simulink model "Prescan_Carsim_0118_cs_old"  (R2019b)
settings: Solver=ode5  StartTime=0.0  StopTime=inf  FixedStep=1/1000  RelTol=1e-3
PreLoadFcn:
  | mbxruntime.callbacks.PreLoadFcn(bdroot);
PostLoadFcn:
  | mbxruntime.callbacks.PostLoadFcn(bdroot);
InitFcn:
  | mbxruntime.callbacks.InitFcn(bdroot);
  | Initialization_Func;
  | %T01_Init_2106;
StartFcn:
  | mbxruntime.callbacks.StartFcn(bdroot);
  | current_sys=gcs;
  | speedblock=Simulink.findBlocks(current_sys,'Name','speed_kmh_Gain');
  | h1=add_exec_event_listener(speedblock,'PostOutputs',@SpeedVisulization);
  | outblock=Simulink.findBlocks(current_sys,'Name','trajectorycurveoutput_Gain');
  | CurveTrajectoryListenerHandle=add_exec_event_listener(outblock,'PostOutputs',@TrajectoryCurve_CallBack);
  | lanedatablock=Simulink.findBlocks(current_sys,'Name','LaneData_Gain');
  | CurveLaneListenerHandle=add_exec_event_listener(lanedatablock,'PostOutputs',@CurveLane_CallBack);
StopFcn:
  | mbxruntime.callbacks.StopFcn(bdroot);
model workspace: external: MAT-File .\Prescan_Carsim_0118_cs_hws.mat (data not in the file)
values from neighbouring files (symbols this model uses):
  g = 9.8    [Initialization_Func.m]
  InitialPlanningParameter = [0,0,1,0,2,2,2,40,60]'    [Initialization_Func.m]
  Kf = 20000    [Initialization_Func.m]
  Kr = 20000    [Initialization_Func.m]
  Lr = 1.644    [Initialization_Func.m]
  M = 1275    [Initialization_Func.m]
  nG = 24    [Initialization_Func.m]
  V = 60/3.6    (= 16.6666666667)    [Initialization_Func.m]
  VehicleBaseLength = Lf+Lr    (= 2.66)    [Initialization_Func.m]
undefined symbols (not defined in the file or in its folder): AAx, AAy, AAz, AVx, AVy, AVz, Ax, Ay, Az, canChannel, DiscIntNeverNeededParam, InitialDPMPDF_Comfort, InitialDPMPDF_Efficiency, InitialDPMPDF_Safety, InitialPDF_DEM, mbxruntime, NormalisedTrajectoryIndicator_Pool, Parameter_Indicator_LookUpTable, Prescan_Carsim_1230_cs_0658e9ca1334a8be, Prescan_Carsim_1230_cs_08c5eb9a1bd7376a, Prescan_Carsim_1230_cs_6cfd759b89b9fc85, Prescan_Carsim_1230_cs_9435cc1cceb5050d, Prescan_Carsim_1230_cs_ac716d34d49f74ab, Prescan_Carsim_1230_cs_be02757d7f212dd5, Rational_Coefficient_Learning, SteeringWheel, TrajectoryIndicatorRange, Vx, Vy, Vz, WheelL0, WheelL1, WheelR0, WheelR1
libraries: canmsglib x11, dsparch4 x6, canlib x3, PreScanSimulinkLibrary x3, Solver_SF x1, autolibshared x1
(part 3 of 8)

== system Prescan_Carsim_0118_cs_old/BMW_X5_SUV_1/Connect The Target /simplefilter ==
  In1 : Inport
  Add : Sum
  Gain : Gain  Gain=0.5
  Memory : Memory
  Out1 : Outport  VectorParamsAs1DForOutWhenUnconnected=off
  wires:
  Gain/1 -> Out1/1
  Memory/1 -> Add/2
  Add/1 -> Gain/1
  In1/1 -> Memory/1, Add/1

== system Prescan_Carsim_0118_cs_old/BMW_X5_SUV_1/DEM updating and Preference Estimation/UpdateDEM ==
  FeedBack_FromDriver : Inport
  TrajectoryIndicator : Inport  Port=2
  Trigger : TriggerPort  TriggerType=either  VariantControl=Variant  PortDimensions=1
  Constant1 : Constant  Value=InitialPDF_DEM
      settings: AttributesFormatString=|
      | The Initial probability density Distribution
      | of the S-C-E weight of the DEM
  Constant2 : Constant  Value=InitialDPMPDF_Safety
      settings: AttributesFormatString=|
      | The Initial probability density Distribution
      | of the DPM for S-C-E
  Constant5 : Constant  Value=InitialDPMPDF_Comfort
      settings: AttributesFormatString=|
      | The Initial probability density Distribution
      | of the DPM for S-C-E
  Constant6 : Constant  Value=InitialDPMPDF_Efficiency
      settings: AttributesFormatString=|
      | The Initial probability density Distribution
      | of the DPM for S-C-E
  Construct Comparison Group : Subsystem
  Online DEM updating : Subsystem
  Trajectory Planning Parameter Management1 : Subsystem  Commented=on
  Trajectory Planning Parameter Management2 : Subsystem
  online DPM building preference estimation accordign to feedback : Subsystem  Commented=on
  PlanningParameter : Outport  InitialOutput=InitialPlanningParameter
  Expected_QueryID : Outport  Port=2
  wires:
  Construct Comparison Group/1(FeedBack) -> Online DEM updating/1(FeedBack)
  online DPM building preference estimation accordign to feedback/1(Expected_TrajectoryIndicators) -> Trajectory Planning Parameter Management1/1(Expected_TrajectoryIndicators)
  online DPM building preference estimation accordign to feedback/2(ExpectedNext_QueryID) -> Trajectory Planning Parameter Management1/2(ExpectedNext_QueryID)
  Trajectory Planning Parameter Management2/1(Trajectory parameter) -> PlanningParameter/1
  Online DEM updating/1(Next_ExpectedTrajectoryIndicator) -> Trajectory Planning Parameter Management2/1(Expected_TrajectoryIndicators)
  Construct Comparison Group/2(Query_Normalized) -> Online DEM updating/2(Query_Compare)
  Constant2/1 -> Online DEM updating/4(PriorDPMPDF_Safety)
  Constant1/1 -> Online DEM updating/3(PriorPDF_DEM)
  Constant6/1 -> Online DEM updating/6(PriorDPMPDF_Efficiency)
  Online DEM updating/2(Next_ExpectedTrajectoryID) -> Trajectory Planning Parameter Management2/2(Next_ExpectedTrajectoryIndicatorID), Expected_QueryID/1
  Constant5/1 -> Online DEM updating/5(PriorDPMPDF_Comfort)
  Construct Comparison Group/3(Evaluated_NormlisedTrajectoryIndicator) -> Online DEM updating/7(Evaluated_Normalised)
  Construct Comparison Group/4(LastPreference_Normalised) -> Online DEM updating/8(LastPreference_NormalisedTrajectoryIndicator)
  FeedBack_FromDriver/1 -> Construct Comparison Group/1(FeedBack_FromDriver)
  TrajectoryIndicator/1 -> Construct Comparison Group/2(TrajectoryIndicator)

== system Prescan_Carsim_0118_cs_old/BMW_X5_SUV_1/DriverFeedBack/Generate the FeedBack Obtainment Trigger Signal ==
  CurveFlag : Inport
  Add : Sum  Inputs=-+
  Clock : Clock
  ConsideringTime (s) : Constant  Value=2
  Relational Operator : RelationalOperator  Operator=>  OutDataTypeStr=boolean  RndMeth=Simplest
  Subsystem : Subsystem
  Trigger Signal of Feedback obtainement : Outport
  wires:
  ConsideringTime (s)/1 -> Relational Operator/2
  Add/1 -> Relational Operator/1  "CurveTime"
  Clock/1 -> Add/2, Subsystem/1(In1)
  Subsystem/1(Beginning Time) -> Add/1
  CurveFlag/1 -> Subsystem/Trigger
  Relational Operator/1 -> Trigger Signal of Feedback obtainement/1

== system Prescan_Carsim_0118_cs_old/BMW_X5_SUV_1/DriverFeedBack/driver evaluation model ==
  TrajectoryIndicators : Inport
  Trigger : TriggerPort  VariantControl=Variant  PortDimensions=1
  Constant : Constant
      settings: AttributesFormatString=|
      | 1: "complete_rational"
      | 2: "probability_rational"
      | 3: "bound_rational"
  RationalCoefficient_Sim : Constant  Value=5
  Scope : Scope
  SimPreferenceDPM_Comfort : Constant  Value=[1,1]
  SimPreferenceDPM_Efficiency : Constant  Value=[1,1]
  SimPreferenceDPM_Safety : Constant  Value=[1,1]
  SimPreference_DEM : Constant  Value=[0.3,0.4,0.3]
  Simulated Driver : MATLAB Function  TreatAsAtomicUnit=on
  feedback : Outport
      settings: AttributesFormatString=|
      | 0: There is no comparison
      | 1: Prefer the former one
      | 2：Prefer the latter one
      | 3: No obvious preference
  FeedBack_Trigger : Outport  Port=2
  wires:
  Simulated Driver/1(Compare_Result) -> feedback/1
  Simulated Driver/3(mis_answered_ind) -> Scope/1
  SimPreference_DEM/1 -> Simulated Driver/2(Preference_DEM)
  SimPreferenceDPM_Safety/1 -> Simulated Driver/3(PreferenceDPM_Safety)
  SimPreferenceDPM_Comfort/1 -> Simulated Driver/4(PreferenceDPM_Comfort)
  SimPreferenceDPM_Efficiency/1 -> Simulated Driver/5(PreferenceDPM_Efficiency)
  RationalCoefficient_Sim/1 -> Simulated Driver/6(Rational_coefficient)
  Constant/1 -> Simulated Driver/7(Driver_Type)
  TrajectoryIndicators/1 -> Simulated Driver/1(TrajectoryIndicator)
  Simulated Driver/2(FeedBack_Count) -> FeedBack_Trigger/1

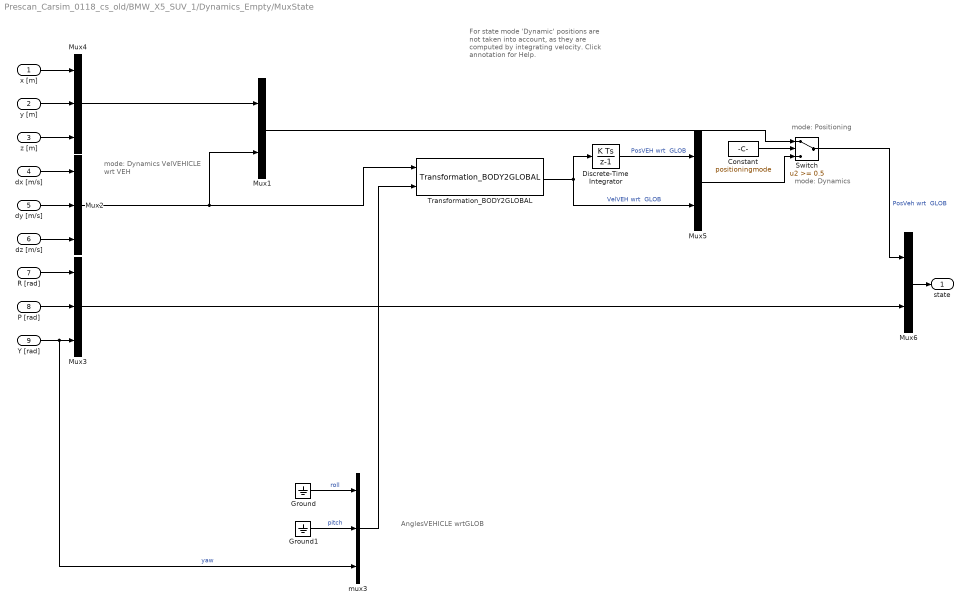
== system Prescan_Carsim_0118_cs_old/BMW_X5_SUV_1/Dynamics_Empty/MuxState ==
  note: mode: Dynamics
  note: mode: Positioning
  note: mode: Dynamics
      | VelVEHICLE
      | wrt VEH
  note: AnglesVEHICLE
      | wrtGLOB
  note: For state mode 'Dynamic' positions
      | are not taken into account, as they
      | are computed by integrating velocity.
      | Click annotation for Help.
  x [m] : Inport  SampleTime=TimeStep
  y [m] : Inport  Port=2  SampleTime=TimeStep
  z [m] : Inport  Port=3  SampleTime=TimeStep
  dx [m/s] : Inport  Port=4  SampleTime=TimeStep
  dy [m/s] : Inport  Port=5  SampleTime=TimeStep
  dz [m/s] : Inport  Port=6  SampleTime=TimeStep
  R [rad] : Inport  Port=7  SampleTime=TimeStep
  P [rad] : Inport  Port=8  SampleTime=TimeStep
  Y [rad] : Inport  Port=9  SampleTime=TimeStep
  Constant : Constant  DisableCoverage=on  Value=positioningmode
  Discrete-Time Integrator : DiscreteIntegrator  SampleTime=TimeStep  ICPrevOutput=DiscIntNeverNeededParam  ICPrevScaledInput=DiscIntNeverNeededParam
  Ground : Ground
  Ground1 : Ground
  Mux1 : Mux  Inputs=[3 3]
  Mux2 : Mux  Inputs=3
  Mux3 : Mux  Inputs=3
  Mux4 : Mux  Inputs=3
  Mux5 : Mux  Inputs=[3 3]
  Mux6 : Mux  Inputs=[6 3]
  Switch : Switch  Threshold=0.5
  Transformation_BODY2GLOBAL : PreScanSimulinkLibrary/Simple_Vehicle_Dynamics/Chassis/MuxDynState/Transformation_BODY2GLOBAL  SystemSampleTime=-1  Latency=0  AutoFrameSizeCalculation=off
  mux3 : Mux  Inputs=3
  state : Outport
  wires:
  Constant/1 -> Switch/2
  Mux6/1 -> state/1
  Mux4/1 -> Mux1/1
  Mux5/1 -> Switch/3
  Mux1/1 -> Switch/1
  Switch/1 -> Mux6/1  "PosVeh wrt  GLOB"
  P [rad]/1 -> Mux3/2
  R [rad]/1 -> Mux3/1
  dz [m/s]/1 -> Mux2/3
  dy [m/s]/1 -> Mux2/2
  dx [m/s]/1 -> Mux2/1
  z [m]/1 -> Mux4/3
  y [m]/1 -> Mux4/2
  x [m]/1 -> Mux4/1
  Ground1/1 -> mux3/2  "pitch"
  Y [rad]/1 -> mux3/3, Mux3/3  "yaw"
  Mux3/1 -> Mux6/2
  Transformation_BODY2GLOBAL/1 -> Discrete-Time Integrator/1, Mux5/2  "VelVEH wrt  GLOB"
  mux3/1 -> Transformation_BODY2GLOBAL/2
  Ground/1 -> mux3/1  "roll"
  Mux2/1 -> Mux1/2, Transformation_BODY2GLOBAL/1
  Discrete-Time Integrator/1 -> Mux5/1  "PosVEH wrt  GLOB"

== system Prescan_Carsim_0118_cs_old/BMW_X5_SUV_1/Dynamics_Empty/STATE_BMW_X5_SUV_1 ==
  State : Inport  SampleTime=TimeStep
  Bus Creator : BusCreator  Inputs=15  OutDataTypeStr=Bus: PRESCAN_STATEACTUATORDATA  NonVirtualBus=on
  Constant : Constant  Value=0
  Demux : Demux  Outputs=15
  Mux : Mux  Inputs=3
  Mux1 : Mux  Inputs=3
  Mux2 : Mux  Inputs=3
  iniBODYAngles wrtVEH [rad] : Constant  Value=Roll0  SampleTime=TimeStep
  iniBODYAngles wrtVEH [rad]1 : Constant  Value=Pitch0  SampleTime=TimeStep
  iniVEHAngles wrtGLOB [rad] : Constant  Value=Yaw0  SampleTime=TimeStep
  iniVEHposition wrtGLOB [m] : Constant  Value=x0  SampleTime=TimeStep
  iniVEHposition wrtGLOB [m]1 : Constant  Value=y0  SampleTime=TimeStep
  iniVEHposition wrtGLOB [m]2 : Constant  Value=z0  SampleTime=TimeStep
  state2FullState : PreScanSimulinkLibrary/state2FullState  SystemSampleTime=-1  Latency=0  AutoFrameSizeCalculation=off
  StateBus : Outport  OutDataTypeStr=Bus: PRESCAN_STATEACTUATORDATA
  wires:
  Mux2/1 -> state2FullState/4
  iniVEHAngles wrtGLOB [rad]/1 -> Mux2/3
  Mux1/1 -> state2FullState/3
  Constant/1 -> Mux2/1, Mux2/2, Mux1/3
  iniBODYAngles wrtVEH [rad]1/1 -> Mux1/2
  iniBODYAngles wrtVEH [rad]/1 -> Mux1/1
  Mux/1 -> state2FullState/2
  iniVEHposition wrtGLOB [m]2/1 -> Mux/3
  iniVEHposition wrtGLOB [m]/1 -> Mux/1
  iniVEHposition wrtGLOB [m]1/1 -> Mux/2
  Demux/15 -> Bus Creator/15  "AngularVelocityYaw"
  Demux/14 -> Bus Creator/14  "AngularVelocityPitch"
  Demux/13 -> Bus Creator/13  "AngularVelocityRoll"
  Demux/12 -> Bus Creator/12  "OrientationYaw"
  Demux/11 -> Bus Creator/11  "OrientationPitch"
  Demux/10 -> Bus Creator/10  "OrientationRoll"
  Demux/9 -> Bus Creator/9  "AccelerationZ"
  Demux/8 -> Bus Creator/8  "AccelerationY"
  Demux/7 -> Bus Creator/7  "AccelerationX"
  Demux/6 -> Bus Creator/6  "VelocityZ"
  Demux/5 -> Bus Creator/5  "VelocityY"
  Demux/4 -> Bus Creator/4  "VelocityX"
  Demux/3 -> Bus Creator/3  "PositionZ"
  Demux/2 -> Bus Creator/2  "PositionY"
  Demux/1 -> Bus Creator/1  "PositionX"
  state2FullState/1 -> Demux/1
  State/1 -> state2FullState/1
  Bus Creator/1 -> StateBus/1

== system Prescan_Carsim_0118_cs_old/BMW_X5_SUV_1/SELF_Demux/compas converter ==
  rotz [rad] : Inport
  cart2compas : Subsystem
  rad2deg : Gain  Gain=180/pi
  heading [deg] : Outport
  wires:
  rad2deg/1 -> cart2compas/1(Angle [deg])
  rotz [rad]/1 -> rad2deg/1
  cart2compas/1(heading [deg]) -> heading [deg]/1

== system Prescan_Carsim_0118_cs_old/BMW_X5_SUV_1/Tracking Control & vehicle dynamics/Lane Keeping Assistance ==
  note: Trajectory Trackin-LQR controller, Carsim Model
  note: Trajectory Trackin-LQR controller, Simulink VDM
  note: Trajectory Tracking Controller-SMC controller
  DataUsedForTracking (PrescanToTarget)t : Inport
  Bus Selector : BusSelector  OutputSignals=Preview Error,HeadError_rad,Curvature,PreviewDistance,Speed_Kmh
  Digital Filter Design6 : dsparch4/Digital Filter Design  Commented=on  mwdsp_browser_bugfix_var=off
  From : From  Commented=on  GotoTag=SMC_c1  TagVisibility=global
  From1 : From  Commented=on  GotoTag=SMC_c2  TagVisibility=global
  From3 : From  Commented=on  GotoTag=delta  TagVisibility=global
  From4 : From  Commented=on  GotoTag=kapa  TagVisibility=global
  Gain : Gain  Gain=180/pi
  Gain1 : Gain  Gain=1/3.6
  Manual Switch : ManualSwitch  CurrentSetting=0
  Manual Switch1 : ManualSwitch  CurrentSetting=0
  Path Tracking - LQR controller : Subsystem  Commented=on
  Path Tracking - LQR controller1 : Subsystem
  Path Tracking - SMC controller : MATLAB Function  Commented=on  TreatAsAtomicUnit=on
  SMC characters : Subsystem  Commented=on
  derivative_filter : Subsystem
  "derivative_filter " : Subsystem
  steering angle_Front(deg) : Outport
  wires:
  Path Tracking - LQR controller/1(SteeringAngle_Front(rad)) -> Manual Switch1/1
  Gain1/1 -> Path Tracking - LQR controller1/7(Speed_m/s), Path Tracking - LQR controller/7(Speed_m/s), Path Tracking - SMC controller/11(v)
  Gain/1 -> steering angle_Front(deg)/1
  "derivative_filter "/1(Out1) -> Path Tracking - LQR controller1/2(PreviewError_dot), Path Tracking - LQR controller/2(PreviewError_dot), Path Tracking - SMC controller/6(PreviewError_dot)
  Digital Filter Design6/1 -> Manual Switch/1  "steering angle"
  From/1 -> Path Tracking - SMC controller/1(c1)
  derivative_filter/1(Out1) -> Path Tracking - LQR controller1/4(HeadingError_dot), Path Tracking - LQR controller/4(HeadingError_dot), Path Tracking - SMC controller/8(HeadingError_dot)
  Path Tracking - SMC controller/1(SteerAngle) -> Digital Filter Design6/1
  From3/1 -> Path Tracking - SMC controller/3(delta)
  From1/1 -> Path Tracking - SMC controller/2(c2)
  From4/1 -> Path Tracking - SMC controller/4(kapa)
  Bus Selector/5 -> Gain1/1  "<Speed_Kmh>"
  Bus Selector/1 -> Path Tracking - SMC controller/5(PreviewError), Path Tracking - LQR controller1/1(PreviewError), Path Tracking - LQR controller/1(PreviewError), "derivative_filter "/1(In1)  "<Preview Error>"
  Bus Selector/4 -> Path Tracking - SMC controller/10(PreviewDistance), Path Tracking - LQR controller1/6(Preview_Distance), Path Tracking - LQR controller/6(Preview_Distance)  "<PreviewDistance>"
  Bus Selector/2 -> Path Tracking - LQR controller1/3(HeadingError), Path Tracking - LQR controller/3(HeadingError), Path Tracking - SMC controller/7(HeadingError), derivative_filter/1(In1)  "<HeadError_rad>"
  Manual Switch/1 -> Gain/1
  Bus Selector/3 -> Path Tracking - LQR controller1/5(Curvature), Path Tracking - LQR controller/5(Curvature), Path Tracking - SMC controller/9(Curvature)  "<Curvature>"
  DataUsedForTracking (PrescanToTarget)t/1 -> Bus Selector/1
  Path Tracking - LQR controller1/1(SteeringAngle_Front(rad)) -> Manual Switch1/2
  Manual Switch1/1 -> Manual Switch/2

== system Prescan_Carsim_0118_cs_old/BMW_X5_SUV_1/Tracking Control & vehicle dynamics/simple_filter10 ==
  In1 : Inport
  Add : Sum
  Gain10 : Gain  Gain=0.5
  Memory : Memory
  Out1 : Outport  VectorParamsAs1DForOutWhenUnconnected=off
  wires:
  Gain10/1 -> Out1/1
  Memory/1 -> Add/2
  In1/1 -> Add/1, Memory/1
  Add/1 -> Gain10/1

== system Prescan_Carsim_0118_cs_old/BMW_X5_SUV_1/Tracking Control & vehicle dynamics/simple_filter11 ==
  In1 : Inport
  Add : Sum
  Gain10 : Gain  Gain=0.5
  Memory : Memory
  Out1 : Outport  VectorParamsAs1DForOutWhenUnconnected=off
  wires:
  Gain10/1 -> Out1/1
  Memory/1 -> Add/2
  In1/1 -> Add/1, Memory/1
  Add/1 -> Gain10/1

== system Prescan_Carsim_0118_cs_old/BMW_X5_SUV_1/Tracking Control & vehicle dynamics/simple_filter6 ==
  In1 : Inport
  Add : Sum
  Gain10 : Gain  Gain=0.5
  Memory : Memory
  Out1 : Outport  VectorParamsAs1DForOutWhenUnconnected=off
  wires:
  Add/1 -> Gain10/1
  In1/1 -> Memory/1, Add/1
  Memory/1 -> Add/2
  Gain10/1 -> Out1/1

== system Prescan_Carsim_0118_cs_old/BMW_X5_SUV_1/Tracking Control & vehicle dynamics/simple_filter7 ==
  In1 : Inport
  Add : Sum
  Gain10 : Gain  Gain=0.5
  Memory : Memory
  Out1 : Outport  VectorParamsAs1DForOutWhenUnconnected=off
  wires:
  Gain10/1 -> Out1/1
  Memory/1 -> Add/2
  In1/1 -> Add/1, Memory/1
  Add/1 -> Gain10/1

== system Prescan_Carsim_0118_cs_old/BMW_X5_SUV_1/Tracking Control & vehicle dynamics/simple_filter8 ==
  In1 : Inport
  Add : Sum
  Gain10 : Gain  Gain=0.5
  Memory : Memory
  Out1 : Outport  VectorParamsAs1DForOutWhenUnconnected=off
  wires:
  Add/1 -> Gain10/1
  In1/1 -> Memory/1, Add/1
  Memory/1 -> Add/2
  Gain10/1 -> Out1/1

== system Prescan_Carsim_0118_cs_old/BMW_X5_SUV_1/Tracking Control & vehicle dynamics/simple_filter9 ==
  In1 : Inport
  Add : Sum
  Gain10 : Gain  Gain=0.5
  Memory : Memory
  Out1 : Outport  VectorParamsAs1DForOutWhenUnconnected=off
  wires:
  Gain10/1 -> Out1/1
  Memory/1 -> Add/2
  In1/1 -> Add/1, Memory/1
  Add/1 -> Gain10/1

== system Prescan_Carsim_0118_cs_old/BMW_X5_SUV_1/Trajectory Indicator Calculation/VehicleInfo_Curve ==
  In1 : Inport
  Trigger : TriggerPort  TriggerType=falling  VariantControl=Variant
  trajectorycurveoutput_Gain : Gain
  VehicleInfo_Curve : Outport
  wires:
  In1/1 -> trajectorycurveoutput_Gain/1
  trajectorycurveoutput_Gain/1 -> VehicleInfo_Curve/1

== system Prescan_Carsim_0118_cs_old/BMW_X5_SUV_1/Trajectory Indicator Calculation/VehicleState_Buffer ==
  In1 : Inport
  Enable : EnablePort  StatesWhenEnabling=reset  PropagateVarSize=During execution
  VehicleInfo_StoreDuringCurve : MATLAB Function  TreatAsAtomicUnit=on
  VehicleInfo_Curve : Outport
  wires:
  In1/1 -> VehicleInfo_StoreDuringCurve/1(VehicleState_Var)
  VehicleInfo_StoreDuringCurve/1(VehicleState_Curve) -> VehicleInfo_Curve/1

== system Prescan_Carsim_0118_cs_old/BMW_X5_SUV_1/VehicleToPrescan/simple_filter10 ==
  In1 : Inport
  Add : Sum
  Gain10 : Gain  Gain=0.5
  Memory : Memory
  Out1 : Outport  VectorParamsAs1DForOutWhenUnconnected=off
  wires:
  Gain10/1 -> Out1/1
  Memory/1 -> Add/2
  In1/1 -> Add/1, Memory/1
  Add/1 -> Gain10/1

== system Prescan_Carsim_0118_cs_old/BMW_X5_SUV_1/VehicleToPrescan/simple_filter11 ==
  In1 : Inport
  Add : Sum
  Gain10 : Gain  Gain=0.5
  Memory : Memory
  Out1 : Outport  VectorParamsAs1DForOutWhenUnconnected=off
  wires:
  Gain10/1 -> Out1/1
  Memory/1 -> Add/2
  In1/1 -> Add/1, Memory/1
  Add/1 -> Gain10/1

== system Prescan_Carsim_0118_cs_old/BMW_X5_SUV_1/VehicleToPrescan/simple_filter6 ==
  In1 : Inport
  Add : Sum
  Gain10 : Gain  Gain=0.5
  Memory : Memory
  Out1 : Outport  VectorParamsAs1DForOutWhenUnconnected=off
  wires:
  Add/1 -> Gain10/1
  In1/1 -> Memory/1, Add/1
  Memory/1 -> Add/2
  Gain10/1 -> Out1/1

== system Prescan_Carsim_0118_cs_old/BMW_X5_SUV_1/VehicleToPrescan/simple_filter7 ==
  In1 : Inport
  Add : Sum
  Gain10 : Gain  Gain=0.5
  Memory : Memory
  Out1 : Outport  VectorParamsAs1DForOutWhenUnconnected=off
  wires:
  Gain10/1 -> Out1/1
  Memory/1 -> Add/2
  In1/1 -> Add/1, Memory/1
  Add/1 -> Gain10/1

== system Prescan_Carsim_0118_cs_old/BMW_X5_SUV_1/VehicleToPrescan/simple_filter8 ==
  In1 : Inport
  Add : Sum
  Gain10 : Gain  Gain=0.5
  Memory : Memory
  Out1 : Outport  VectorParamsAs1DForOutWhenUnconnected=off
  wires:
  Add/1 -> Gain10/1
  In1/1 -> Memory/1, Add/1
  Memory/1 -> Add/2
  Gain10/1 -> Out1/1

== system Prescan_Carsim_0118_cs_old/BMW_X5_SUV_1/VehicleToPrescan/simple_filter9 ==
  In1 : Inport
  Add : Sum
  Gain10 : Gain  Gain=0.5
  Memory : Memory
  Out1 : Outport  VectorParamsAs1DForOutWhenUnconnected=off
  wires:
  Gain10/1 -> Out1/1
  Memory/1 -> Add/2
  In1/1 -> Add/1, Memory/1
  Add/1 -> Gain10/1

== system Prescan_Carsim_0118_cs_old/BMW_X5_SUV_1/WheelDisplacement_Mux/WheelL0_Mux ==
  X [m] : Inport
  Y [m] : Inport  Port=2
  Z [m] : Inport  Port=3
  Roll [rad] : Inport  Port=4
  Pitch [rad] : Inport  Port=5
  Yaw [rad] : Inport  Port=6
  Bus Creator : BusCreator  Inputs=3  OutDataTypeStr=Bus: PRESCAN_XYZ_DATA
  Bus Creator1 : BusCreator  Inputs=3  OutDataTypeStr=Bus: PRESCAN_RPY_DATA
  Bus Creator2 : BusCreator  Inputs=2  OutDataTypeStr=Bus: PRESCAN_POSE_DATA
  Joint : Outport
  wires:
  Yaw [rad]/1 -> Bus Creator1/3  "Yaw"
  Bus Creator1/1 -> Bus Creator2/2  "ORIENTATION"
  Bus Creator/1 -> Bus Creator2/1  "POSITION"
  X [m]/1 -> Bus Creator/1  "X"
  Y [m]/1 -> Bus Creator/2  "Y"
  Z [m]/1 -> Bus Creator/3  "Z"
  Bus Creator2/1 -> Joint/1
  Roll [rad]/1 -> Bus Creator1/1  "Roll"
  Pitch [rad]/1 -> Bus Creator1/2  "Pitch"

== system Prescan_Carsim_0118_cs_old/BMW_X5_SUV_1/WheelDisplacement_Mux/WheelL1_Mux ==
  X [m] : Inport
  Y [m] : Inport  Port=2
  Z [m] : Inport  Port=3
  Roll [rad] : Inport  Port=4
  Pitch [rad] : Inport  Port=5
  Yaw [rad] : Inport  Port=6
  Bus Creator : BusCreator  Inputs=3  OutDataTypeStr=Bus: PRESCAN_XYZ_DATA
  Bus Creator1 : BusCreator  Inputs=3  OutDataTypeStr=Bus: PRESCAN_RPY_DATA
  Bus Creator2 : BusCreator  Inputs=2  OutDataTypeStr=Bus: PRESCAN_POSE_DATA
  Joint : Outport
  wires:
  Yaw [rad]/1 -> Bus Creator1/3  "Yaw"
  Bus Creator1/1 -> Bus Creator2/2  "ORIENTATION"
  Bus Creator/1 -> Bus Creator2/1  "POSITION"
  X [m]/1 -> Bus Creator/1  "X"
  Y [m]/1 -> Bus Creator/2  "Y"
  Z [m]/1 -> Bus Creator/3  "Z"
  Bus Creator2/1 -> Joint/1
  Roll [rad]/1 -> Bus Creator1/1  "Roll"
  Pitch [rad]/1 -> Bus Creator1/2  "Pitch"

== system Prescan_Carsim_0118_cs_old/BMW_X5_SUV_1/WheelDisplacement_Mux/WheelR0_Mux ==
  X [m] : Inport
  Y [m] : Inport  Port=2
  Z [m] : Inport  Port=3
  Roll [rad] : Inport  Port=4
  Pitch [rad] : Inport  Port=5
  Yaw [rad] : Inport  Port=6
  Bus Creator : BusCreator  Inputs=3  OutDataTypeStr=Bus: PRESCAN_XYZ_DATA
  Bus Creator1 : BusCreator  Inputs=3  OutDataTypeStr=Bus: PRESCAN_RPY_DATA
  Bus Creator2 : BusCreator  Inputs=2  OutDataTypeStr=Bus: PRESCAN_POSE_DATA
  Joint : Outport
  wires:
  Yaw [rad]/1 -> Bus Creator1/3  "Yaw"
  Bus Creator1/1 -> Bus Creator2/2  "ORIENTATION"
  Bus Creator/1 -> Bus Creator2/1  "POSITION"
  X [m]/1 -> Bus Creator/1  "X"
  Y [m]/1 -> Bus Creator/2  "Y"
  Z [m]/1 -> Bus Creator/3  "Z"
  Bus Creator2/1 -> Joint/1
  Roll [rad]/1 -> Bus Creator1/1  "Roll"
  Pitch [rad]/1 -> Bus Creator1/2  "Pitch"

== system Prescan_Carsim_0118_cs_old/BMW_X5_SUV_1/WheelDisplacement_Mux/WheelR1_Mux ==
  X [m] : Inport
  Y [m] : Inport  Port=2
  Z [m] : Inport  Port=3
  Roll [rad] : Inport  Port=4
  Pitch [rad] : Inport  Port=5
  Yaw [rad] : Inport  Port=6
  Bus Creator : BusCreator  Inputs=3  OutDataTypeStr=Bus: PRESCAN_XYZ_DATA
  Bus Creator1 : BusCreator  Inputs=3  OutDataTypeStr=Bus: PRESCAN_RPY_DATA
  Bus Creator2 : BusCreator  Inputs=2  OutDataTypeStr=Bus: PRESCAN_POSE_DATA
  Joint : Outport
  wires:
  Yaw [rad]/1 -> Bus Creator1/3  "Yaw"
  Bus Creator1/1 -> Bus Creator2/2  "ORIENTATION"
  Bus Creator/1 -> Bus Creator2/1  "POSITION"
  X [m]/1 -> Bus Creator/1  "X"
  Y [m]/1 -> Bus Creator/2  "Y"
  Z [m]/1 -> Bus Creator/3  "Z"
  Bus Creator2/1 -> Joint/1
  Roll [rad]/1 -> Bus Creator1/1  "Roll"
  Pitch [rad]/1 -> Bus Creator1/2  "Pitch"

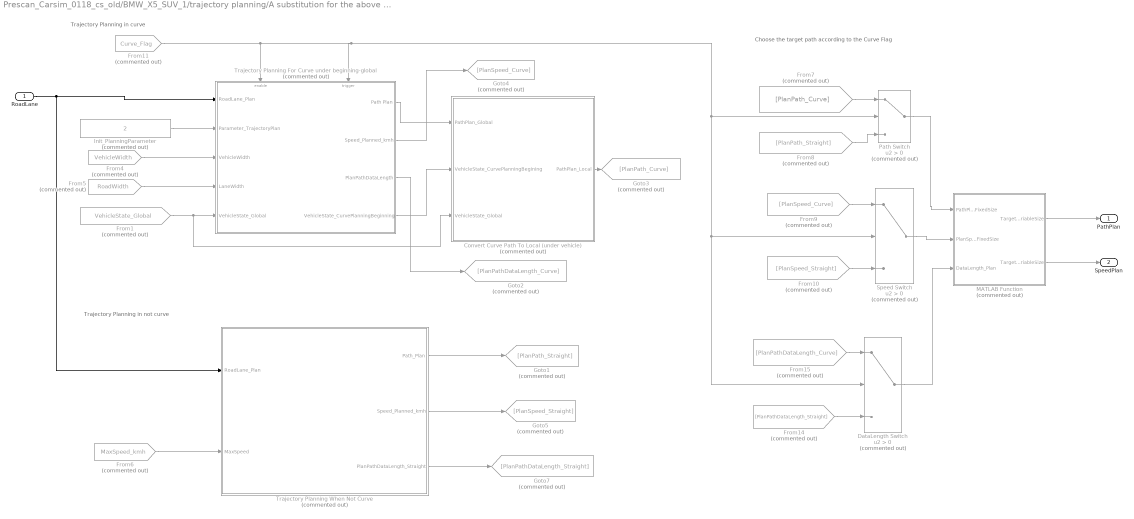
== system Prescan_Carsim_0118_cs_old/BMW_X5_SUV_1/trajectory planning/A substitution for the above trajectory planning subsystem ==
  note: Choose the target path according to the Curve Flag
  note: Trajectory Planning in not curve
  note: Trajectory Planning in curve
  RoadLane : Inport
  Convert Curve Path To Local (under vehicle) : MATLAB Function  Commented=on  TreatAsAtomicUnit=on
  DataLength Switch : Switch  Commented=on  Criteria=u2 > Threshold
  From1 : From  Commented=on  GotoTag=VehicleState_Global  TagVisibility=global
  From10 : From  Commented=on  GotoTag=PlanSpeed_Straight
  From11 : From  Commented=on  GotoTag=Curve_Flag  TagVisibility=global
  From14 : From  Commented=on  GotoTag=PlanPathDataLength_Straight
  From15 : From  Commented=on  GotoTag=PlanPathDataLength_Curve
  From4 : From  Commented=on  GotoTag=VehicleWidth  TagVisibility=global
  From5 : From  Commented=on  GotoTag=RoadWidth  TagVisibility=global
  From6 : From  Commented=on  GotoTag=MaxSpeed_kmh  TagVisibility=global
  From7 : From  Commented=on  GotoTag=PlanPath_Curve
  From8 : From  Commented=on  GotoTag=PlanPath_Straight
  From9 : From  Commented=on  GotoTag=PlanSpeed_Curve
  Goto1 : Goto  Commented=on  GotoTag=PlanPath_Straight
      settings: AttributesFormatString=output:fixed size,1000*2
  Goto2 : Goto  Commented=on  GotoTag=PlanPathDataLength_Curve
  Goto3 : Goto  Commented=on  GotoTag=PlanPath_Curve
      settings: AttributesFormatString=|
      | Path local under the vehicle
      | output:fixed size 1000*2
  Goto4 : Goto  Commented=on  GotoTag=PlanSpeed_Curve
      settings: AttributesFormatString=The size is fixed 1000*1
  Goto5 : Goto  Commented=on  GotoTag=PlanSpeed_Straight
      settings: AttributesFormatString=The size vas fixed 1000*1
  Goto7 : Goto  Commented=on  GotoTag=PlanPathDataLength_Straight
      settings: AttributesFormatString=|
      | Used to extract the valid
      | PlanPath data
  Init_PlanningParameter : Constant  Commented=on  Value=2
  MATLAB Function : MATLAB Function  Commented=on  TreatAsAtomicUnit=on  SystemSampleTime=1/20
      settings: AttributesFormatString=|
      | Convert Variable Size into Fixed Size
      | Specified Sample Time:1/20
  Path Switch : Switch  Commented=on  Criteria=u2 > Threshold
  Speed Switch : Switch  Commented=on  Criteria=u2 > Threshold
  Trajectory Planning For Curve under beginning-global : Subsystem  Commented=on
  Trajectory Planning When Not Curve : MATLAB Function  Commented=on  TreatAsAtomicUnit=on
  PathPlan : Outport
  SpeedPlan : Outport  Port=2
  wires:
  From9/1 -> Speed Switch/1
  From11/1 -> Trajectory Planning For Curve under beginning-global/Trigger, Speed Switch/2, DataLength Switch/2, Path Switch/2, Trajectory Planning For Curve under beginning-global/Enable
  Trajectory Planning For Curve under beginning-global/2(Speed_Planned_kmh) -> Goto4/1
  From15/1 -> DataLength Switch/1
  Path Switch/1 -> MATLAB Function/1(PathPlan_FixedSize)
  DataLength Switch/1 -> MATLAB Function/3(DataLength_Plan)
  From10/1 -> Speed Switch/3
  From14/1 -> DataLength Switch/3
  From8/1 -> Path Switch/3
  Speed Switch/1 -> MATLAB Function/2(PlanSpeed_FixedSize)
  Trajectory Planning When Not Curve/3(PlanPathDataLength_Straight) -> Goto7/1
  Trajectory Planning For Curve under beginning-global/3(PlanPathDataLength) -> Goto2/1
  Trajectory Planning For Curve under beginning-global/1(Path Plan) -> Convert Curve Path To Local (under vehicle)/1(PathPlan_Global)
  From1/1 -> Trajectory Planning For Curve under beginning-global/5(VehicleState_Global), Convert Curve Path To Local (under vehicle)/3(VehicleState_Global)
  Trajectory Planning For Curve under beginning-global/4(VehicleState_CurvePlanningBeginning) -> Convert Curve Path To Local (under vehicle)/2(VehicleState_CurvePlanningBegining)
  Init_PlanningParameter/1 -> Trajectory Planning For Curve under beginning-global/2(Parameter_TrajectoryPlan)
  RoadLane/1 -> Trajectory Planning When Not Curve/1(RoadLane_Plan), Trajectory Planning For Curve under beginning-global/1(RoadLane_Plan)
  Trajectory Planning When Not Curve/2(Speed_Planned_kmh) -> Goto5/1
  From7/1 -> Path Switch/1
  From5/1 -> Trajectory Planning For Curve under beginning-global/4(LaneWidth)
  From4/1 -> Trajectory Planning For Curve under beginning-global/3(VehicleWidth)
  Trajectory Planning When Not Curve/1(Path_Plan) -> Goto1/1
  Convert Curve Path To Local (under vehicle)/1(PathPlan_Local) -> Goto3/1
  From6/1 -> Trajectory Planning When Not Curve/2(MaxSpeed)
  MATLAB Function/1(TargetPath_VariableSize) -> PathPlan/1
  MATLAB Function/2(TargetSpeed_VariableSize) -> SpeedPlan/1

== system Prescan_Carsim_0118_cs_old/BMW_X5_SUV_1/trajectory planning/Generate Road Lane from Polyfit TLC calculation  ==
  RoadLane_Plan : Inport
  PolyRoadLane : Inport  Port=2
  RoadLaneEnd_Rotation : Inport  Port=3
  Mux : Mux  Inputs=3
  Pre_Dis : Constant  Value=150
      settings: AttributesFormatString=The Preview Distance used to calculate the TLC
  Scope : Scope
  Scope1 : Scope
  "TLC calculation and Lane Generation Road Lane " : MATLAB Function  TreatAsAtomicUnit=on
      settings: AttributesFormatString=|
      | The TLC could not be calculated because
      | of the optimal function is not available
      | for simulink code generation
  tag scope: LateralOffset=global, TLC_Left=global, TLC_Right=global
  wires:
  PolyRoadLane/1 -> "TLC calculation and Lane Generation Road Lane "/2(PolyRoadLane)
  "TLC calculation and Lane Generation Road Lane "/2(TLC_Left) -> Mux/1, [TLC_Left]
  [Interval_RoadSegment] -> "TLC calculation and Lane Generation Road Lane "/4(IntervalRoadSegment)
  RoadLaneEnd_Rotation/1 -> "TLC calculation and Lane Generation Road Lane "/3(RoadLaneEnd_Rotation)
  [RoadWidth] -> "TLC calculation and Lane Generation Road Lane "/5(Width_Road)
  [VehicleWidth] -> "TLC calculation and Lane Generation Road Lane "/6(Width_Vehicle)
  Pre_Dis/1 -> "TLC calculation and Lane Generation Road Lane "/8(Range)
  [VehicleBaseLength] -> "TLC calculation and Lane Generation Road Lane "/7(Length_Vehicle)
  [YawRate] -> "TLC calculation and Lane Generation Road Lane "/9(YawRate)
  [Speed_Rel] -> "TLC calculation and Lane Generation Road Lane "/10(Speed)
  "TLC calculation and Lane Generation Road Lane "/3(TLC_Right) -> Mux/2, [TLC_Right]
  "TLC calculation and Lane Generation Road Lane "/1(LateralOffset) -> Scope1/1, [LateralOffset]
  Mux/1 -> Scope/1
  RoadLane_Plan/1 -> "TLC calculation and Lane Generation Road Lane "/1(RoadLanePlan)
  [Curve_Flag] -> Mux/3

== system Prescan_Carsim_0118_cs_old/BMW_X5_SUV_1/trajectory planning/Out of Specific Curve Planning ==
  RoadLane_Plan : Inport
  MaxSpeed_Kmh : Inport  Port=2
  Action Port : ActionPort  ActionPortLabel=else
  Trajectory Planning When Not Curve : MATLAB Function  TreatAsAtomicUnit=on
  Path Plan : Outport
  Speed_Planned_kmh : Outport  Port=2
  PlanPathDataLength : Outport  Port=3
  wires:
  RoadLane_Plan/1 -> Trajectory Planning When Not Curve/1(RoadLane_Plan)
  Trajectory Planning When Not Curve/1(Path_Plan) -> Path Plan/1
  Trajectory Planning When Not Curve/2(Speed_Planned_kmh) -> Speed_Planned_kmh/1
  Trajectory Planning When Not Curve/3(PlanPathDataLength_Straight) -> PlanPathDataLength/1
  MaxSpeed_Kmh/1 -> Trajectory Planning When Not Curve/2(MaxSpeed)

== system Prescan_Carsim_0118_cs_old/BMW_X5_SUV_1/trajectory planning/Specific Curve Trajectory Planning ==
  CurveFlag : Inport
  RoadLane_Plan : Inport  Port=2
  PlanningParameter : Inport  Port=3
  VehicleWidth : Inport  Port=4
  LaneWidth : Inport  Port=5
  VehicleState_Global : Inport  Port=6
  Action Port : ActionPort  InitializeStates=reset  PropagateVarSize=During execution  ActionPortLabel=if(u1 > 0)
  Convert Curve Path To Local (under vehicle) : MATLAB Function  TreatAsAtomicUnit=on
  Trajectory Planning For Curve under beginning-global : Subsystem
  Path Plan : Outport
  Speed_Planned_kmh : Outport  Port=2
  PlanPathDataLength : Outport  Port=3
  wires:
  CurveFlag/1 -> Trajectory Planning For Curve under beginning-global/Trigger
  Trajectory Planning For Curve under beginning-global/1(Path Plan) -> Convert Curve Path To Local (under vehicle)/1(PathPlan_Global)
  Convert Curve Path To Local (under vehicle)/1(PathPlan_Local) -> Path Plan/1
  Trajectory Planning For Curve under beginning-global/2(Speed_Planned_kmh) -> Speed_Planned_kmh/1
  Trajectory Planning For Curve under beginning-global/3(PlanPathDataLength) -> PlanPathDataLength/1
  RoadLane_Plan/1 -> Trajectory Planning For Curve under beginning-global/1(RoadLane_Plan)
  VehicleState_Global/1 -> Trajectory Planning For Curve under beginning-global/5(VehicleState_Global), Convert Curve Path To Local (under vehicle)/2(VehicleState_Global)
  VehicleWidth/1 -> Trajectory Planning For Curve under beginning-global/3(VehicleWidth)
  LaneWidth/1 -> Trajectory Planning For Curve under beginning-global/4(LaneWidth)
  PlanningParameter/1 -> Trajectory Planning For Curve under beginning-global/2(Parameter_TrajectoryPlan)

== system Prescan_Carsim_0118_cs_old/BMW_X5_SUV_1/trajectory planning/Subsystem ==
  Choose curve length for different curve No : MultiPortSwitch  Inputs=4  DataPortForDefault=Additional data port  DiagnosticForDefault=None
  Constant : Constant
  Constant1 : Constant  Value=0
  "Curve 1 " : Constant  Value=308
  Curve 2 : Constant  Value=308
  Curve 3 : Constant  Value=308
  Curve 4 : Constant  Value=308
  Determination of Curve Road No : Subsystem
  Not Curve : Constant  Value=160
  Sum : Sum  Inputs=2
  Switch : Switch  Criteria=u2 > Threshold  Threshold=0.5
  The planned path length after curve : Constant  Value=8
      settings: AttributesFormatString=Should consider the Preview Distance
  Expected PathPlanning Length : Outport
  Curve Flag : Outport  Port=2
      settings: AttributesFormatString=|
      | 1: Curve
      | 0: Not Curve
  wires:
  Determination of Curve Road No/1(Curve No) -> Switch/2, Choose curve length for different curve No/1
  Not Curve/1 -> Choose curve length for different curve No/6
  Curve 4/1 -> Choose curve length for different curve No/5
  Curve 3/1 -> Choose curve length for different curve No/4
  Sum/1 -> Expected PathPlanning Length/1
  Curve 2/1 -> Choose curve length for different curve No/3
  "Curve 1 "/1 -> Choose curve length for different curve No/2
  The planned path length after curve/1 -> Sum/2
  Choose curve length for different curve No/1 -> Sum/1
  Switch/1 -> Curve Flag/1
  Constant/1 -> Switch/1
  Constant1/1 -> Switch/3

== system Prescan_Carsim_0118_cs_old/SteeringWheel_pivot_BMW_X5_SUV_1/Actuator/visu_Rotate ==
  In1 : Inport
  sfun_RPYActuator : S-Function  FunctionName=sfun_RPYActuator  Parameters=SParameter1, SParameter2, SampleTime  SFunctionDeploymentMode=off  EnableBusSupport=off  mask(Legacy Function){SFunctionSpec=void prescan_outputFcn(void ** work1,  PRESCAN_XYZ_DATA u1[1]), SParameter1=UniqueID, SParameter2=uint8([Object3DID 0]), SampleTime=TimeStep, ShowSpec=on}
      mask prompts: SParameter1 "P1:"; SParameter2 "P2:"; SampleTime "Sample time (-1 for inherited):"; ShowSpec "Display function specification"
      mask help:
      | This block allows you to call the legacy functions specified by the following Legacy Code Tool definition:
      | def.SFunctionName = 'sfun_PositionActuator';
      | def.OutputFcnSpec = 'void prescan_outputFcn(void ** work1,  PRESCAN_XYZ_DATA u1[1])';
      | def.StartFcnSpec = 'void prescan_startFcn(void ** work1, uint8 p1[], double p2)';
      | def.TerminateFcnSpec = 'void prescan_terminateFcn(void ** work1)';
      | def.HeaderFiles = {'prescan_positionactuator_data.h', 'prescan_header_data.h', 'prescan_SFunLibrary.h', 'prescan_CreateLogHandler.h', 'prescan_CreateErrorHandler.h'};
      | def.SourceFiles = {'prescan_MexLogHandler.cpp', 'prescan_SimStructErrorHandler.cpp', 'prescan_ConcurrentLogHandler.cpp', 'prescan_ConcurrentErrorHandler.cpp'};
      | def.HostLibFiles = {'sensorinterfaced.lib'};
      | def.TargetLibFiles = {'sensorinterfaced.so'};
      | def.IncPaths = {'.', 'C:\prescandev\vislibrary\vis\..\pimp\include\sensors\InterfaceRTW'};
      | def.SrcPaths = {'.'};
      | def.LibPaths = {'C:\\prescandev\\vislibrary_build\lib'};
      | def.SampleTime = 'parameterized';
      mask Help: <p>This block was generated automatically by the Legacy Code Tool. For detailed help on this tool, call<a href="matlab:legacy_code('help')"> legacy_code('help')</a>.</p>
      mask Callback ShowSpec:
      | if strcmp(get_param(gcbh, 'ShowSpec'), 'on')
      |   set_param(gcbh, 'MaskDisplay', sprintf('fprintf(''%s'');', get_param(gcbh, 'SFunctionSpec')));
      | else
      |   set_param(gcbh, 'MaskDisplay', sprintf('fprintf(''%s'');', get_param(gcbh, 'FunctionName')));
      | end
      mask Display: fprintf('void prescan_outputFcn(void ** work1,  PRESCAN_XYZ_DATA u1[1])');
  wires:
  In1/1 -> sfun_RPYActuator/1

== system Prescan_Carsim_0118_cs_old/SteeringWheel_pivot_BMW_X5_SUV_1/Actuator/visu_Translate ==
  In1 : Inport
  sfun_PositionActuator : S-Function  FunctionName=sfun_PositionActuator  Parameters=SParameter1, SParameter2, SampleTime  SFunctionDeploymentMode=off  EnableBusSupport=off  mask(Legacy Function){SFunctionSpec=void prescan_outputFcn(void ** work1,  PRESCAN_XYZ_DATA u1[1]), SParameter1=uint8([Object3DID 0]), SParameter2=UniqueID, SampleTime=TimeStep, ShowSpec=on}
      mask prompts: SParameter1 "P1:"; SParameter2 "P2:"; SampleTime "Sample time (-1 for inherited):"; ShowSpec "Display function specification"
      mask help:
      | This block allows you to call the legacy functions specified by the following Legacy Code Tool definition:
      | def.SFunctionName = 'sfun_PositionActuator';
      | def.OutputFcnSpec = 'void prescan_outputFcn(void ** work1,  PRESCAN_XYZ_DATA u1[1])';
      | def.StartFcnSpec = 'void prescan_startFcn(void ** work1, uint8 p1[], double p2)';
      | def.TerminateFcnSpec = 'void prescan_terminateFcn(void ** work1)';
      | def.HeaderFiles = {'prescan_positionactuator_data.h', 'prescan_header_data.h', 'prescan_SFunLibrary.h', 'prescan_CreateLogHandler.h', 'prescan_CreateErrorHandler.h'};
      | def.SourceFiles = {'prescan_MexLogHandler.cpp', 'prescan_SimStructErrorHandler.cpp', 'prescan_ConcurrentLogHandler.cpp', 'prescan_ConcurrentErrorHandler.cpp'};
      | def.HostLibFiles = {'sensorinterfaced.lib'};
      | def.TargetLibFiles = {'sensorinterfaced.so'};
      | def.IncPaths = {'.', 'C:\prescandev\vislibrary\vis\..\pimp\include\sensors\InterfaceRTW'};
      | def.SrcPaths = {'.'};
      | def.LibPaths = {'C:\\prescandev\\vislibrary_build\lib'};
      | def.SampleTime = 'parameterized';
      mask Help: <p>This block was generated automatically by the Legacy Code Tool. For detailed help on this tool, call<a href="matlab:legacy_code('help')"> legacy_code('help')</a>.</p>
      mask Callback ShowSpec:
      | if strcmp(get_param(gcbh, 'ShowSpec'), 'on')
      |   set_param(gcbh, 'MaskDisplay', sprintf('fprintf(''%s'');', get_param(gcbh, 'SFunctionSpec')));
      | else
      |   set_param(gcbh, 'MaskDisplay', sprintf('fprintf(''%s'');', get_param(gcbh, 'FunctionName')));
      | end
      mask Display: fprintf('void prescan_outputFcn(void ** work1,  PRESCAN_XYZ_DATA u1[1])');
  wires:
  In1/1 -> sfun_PositionActuator/1

== system Prescan_Carsim_0118_cs_old/WheelL0_BMW_X5_SUV_1/Actuator/visu_Rotate ==
  In1 : Inport
  sfun_RPYActuator : S-Function  FunctionName=sfun_RPYActuator  Parameters=SParameter1, SParameter2, SampleTime  SFunctionDeploymentMode=off  EnableBusSupport=off  mask(Legacy Function){SFunctionSpec=void prescan_outputFcn(void ** work1,  PRESCAN_XYZ_DATA u1[1]), SParameter1=UniqueID, SParameter2=uint8([Object3DID 0]), SampleTime=TimeStep, ShowSpec=on}
      mask prompts: SParameter1 "P1:"; SParameter2 "P2:"; SampleTime "Sample time (-1 for inherited):"; ShowSpec "Display function specification"
      mask help:
      | This block allows you to call the legacy functions specified by the following Legacy Code Tool definition:
      | def.SFunctionName = 'sfun_PositionActuator';
      | def.OutputFcnSpec = 'void prescan_outputFcn(void ** work1,  PRESCAN_XYZ_DATA u1[1])';
      | def.StartFcnSpec = 'void prescan_startFcn(void ** work1, uint8 p1[], double p2)';
      | def.TerminateFcnSpec = 'void prescan_terminateFcn(void ** work1)';
      | def.HeaderFiles = {'prescan_positionactuator_data.h', 'prescan_header_data.h', 'prescan_SFunLibrary.h', 'prescan_CreateLogHandler.h', 'prescan_CreateErrorHandler.h'};
      | def.SourceFiles = {'prescan_MexLogHandler.cpp', 'prescan_SimStructErrorHandler.cpp', 'prescan_ConcurrentLogHandler.cpp', 'prescan_ConcurrentErrorHandler.cpp'};
      | def.HostLibFiles = {'sensorinterfaced.lib'};
      | def.TargetLibFiles = {'sensorinterfaced.so'};
      | def.IncPaths = {'.', 'C:\prescandev\vislibrary\vis\..\pimp\include\sensors\InterfaceRTW'};
      | def.SrcPaths = {'.'};
      | def.LibPaths = {'C:\\prescandev\\vislibrary_build\lib'};
      | def.SampleTime = 'parameterized';
      mask Help: <p>This block was generated automatically by the Legacy Code Tool. For detailed help on this tool, call<a href="matlab:legacy_code('help')"> legacy_code('help')</a>.</p>
      mask Callback ShowSpec:
      | if strcmp(get_param(gcbh, 'ShowSpec'), 'on')
      |   set_param(gcbh, 'MaskDisplay', sprintf('fprintf(''%s'');', get_param(gcbh, 'SFunctionSpec')));
      | else
      |   set_param(gcbh, 'MaskDisplay', sprintf('fprintf(''%s'');', get_param(gcbh, 'FunctionName')));
      | end
      mask Display: fprintf('void prescan_outputFcn(void ** work1,  PRESCAN_XYZ_DATA u1[1])');
  wires:
  In1/1 -> sfun_RPYActuator/1

== system Prescan_Carsim_0118_cs_old/WheelL0_BMW_X5_SUV_1/Actuator/visu_Translate ==
  In1 : Inport
  sfun_PositionActuator : S-Function  FunctionName=sfun_PositionActuator  Parameters=SParameter1, SParameter2, SampleTime  SFunctionDeploymentMode=off  EnableBusSupport=off  mask(Legacy Function){SFunctionSpec=void prescan_outputFcn(void ** work1,  PRESCAN_XYZ_DATA u1[1]), SParameter1=uint8([Object3DID 0]), SParameter2=UniqueID, SampleTime=TimeStep, ShowSpec=on}
      mask prompts: SParameter1 "P1:"; SParameter2 "P2:"; SampleTime "Sample time (-1 for inherited):"; ShowSpec "Display function specification"
      mask help:
      | This block allows you to call the legacy functions specified by the following Legacy Code Tool definition:
      | def.SFunctionName = 'sfun_PositionActuator';
      | def.OutputFcnSpec = 'void prescan_outputFcn(void ** work1,  PRESCAN_XYZ_DATA u1[1])';
      | def.StartFcnSpec = 'void prescan_startFcn(void ** work1, uint8 p1[], double p2)';
      | def.TerminateFcnSpec = 'void prescan_terminateFcn(void ** work1)';
      | def.HeaderFiles = {'prescan_positionactuator_data.h', 'prescan_header_data.h', 'prescan_SFunLibrary.h', 'prescan_CreateLogHandler.h', 'prescan_CreateErrorHandler.h'};
      | def.SourceFiles = {'prescan_MexLogHandler.cpp', 'prescan_SimStructErrorHandler.cpp', 'prescan_ConcurrentLogHandler.cpp', 'prescan_ConcurrentErrorHandler.cpp'};
      | def.HostLibFiles = {'sensorinterfaced.lib'};
      | def.TargetLibFiles = {'sensorinterfaced.so'};
      | def.IncPaths = {'.', 'C:\prescandev\vislibrary\vis\..\pimp\include\sensors\InterfaceRTW'};
      | def.SrcPaths = {'.'};
      | def.LibPaths = {'C:\\prescandev\\vislibrary_build\lib'};
      | def.SampleTime = 'parameterized';
      mask Help: <p>This block was generated automatically by the Legacy Code Tool. For detailed help on this tool, call<a href="matlab:legacy_code('help')"> legacy_code('help')</a>.</p>
      mask Callback ShowSpec:
      | if strcmp(get_param(gcbh, 'ShowSpec'), 'on')
      |   set_param(gcbh, 'MaskDisplay', sprintf('fprintf(''%s'');', get_param(gcbh, 'SFunctionSpec')));
      | else
      |   set_param(gcbh, 'MaskDisplay', sprintf('fprintf(''%s'');', get_param(gcbh, 'FunctionName')));
      | end
      mask Display: fprintf('void prescan_outputFcn(void ** work1,  PRESCAN_XYZ_DATA u1[1])');
  wires:
  In1/1 -> sfun_PositionActuator/1

== system Prescan_Carsim_0118_cs_old/WheelL1_BMW_X5_SUV_1/Actuator/visu_Rotate ==
  In1 : Inport
  sfun_RPYActuator : S-Function  FunctionName=sfun_RPYActuator  Parameters=SParameter1, SParameter2, SampleTime  SFunctionDeploymentMode=off  EnableBusSupport=off  mask(Legacy Function){SFunctionSpec=void prescan_outputFcn(void ** work1,  PRESCAN_XYZ_DATA u1[1]), SParameter1=UniqueID, SParameter2=uint8([Object3DID 0]), SampleTime=TimeStep, ShowSpec=on}
      mask prompts: SParameter1 "P1:"; SParameter2 "P2:"; SampleTime "Sample time (-1 for inherited):"; ShowSpec "Display function specification"
      mask help:
      | This block allows you to call the legacy functions specified by the following Legacy Code Tool definition:
      | def.SFunctionName = 'sfun_PositionActuator';
      | def.OutputFcnSpec = 'void prescan_outputFcn(void ** work1,  PRESCAN_XYZ_DATA u1[1])';
      | def.StartFcnSpec = 'void prescan_startFcn(void ** work1, uint8 p1[], double p2)';
      | def.TerminateFcnSpec = 'void prescan_terminateFcn(void ** work1)';
      | def.HeaderFiles = {'prescan_positionactuator_data.h', 'prescan_header_data.h', 'prescan_SFunLibrary.h', 'prescan_CreateLogHandler.h', 'prescan_CreateErrorHandler.h'};
      | def.SourceFiles = {'prescan_MexLogHandler.cpp', 'prescan_SimStructErrorHandler.cpp', 'prescan_ConcurrentLogHandler.cpp', 'prescan_ConcurrentErrorHandler.cpp'};
      | def.HostLibFiles = {'sensorinterfaced.lib'};
      | def.TargetLibFiles = {'sensorinterfaced.so'};
      | def.IncPaths = {'.', 'C:\prescandev\vislibrary\vis\..\pimp\include\sensors\InterfaceRTW'};
      | def.SrcPaths = {'.'};
      | def.LibPaths = {'C:\\prescandev\\vislibrary_build\lib'};
      | def.SampleTime = 'parameterized';
      mask Help: <p>This block was generated automatically by the Legacy Code Tool. For detailed help on this tool, call<a href="matlab:legacy_code('help')"> legacy_code('help')</a>.</p>
      mask Callback ShowSpec:
      | if strcmp(get_param(gcbh, 'ShowSpec'), 'on')
      |   set_param(gcbh, 'MaskDisplay', sprintf('fprintf(''%s'');', get_param(gcbh, 'SFunctionSpec')));
      | else
      |   set_param(gcbh, 'MaskDisplay', sprintf('fprintf(''%s'');', get_param(gcbh, 'FunctionName')));
      | end
      mask Display: fprintf('void prescan_outputFcn(void ** work1,  PRESCAN_XYZ_DATA u1[1])');
  wires:
  In1/1 -> sfun_RPYActuator/1

== system Prescan_Carsim_0118_cs_old/WheelL1_BMW_X5_SUV_1/Actuator/visu_Translate ==
  In1 : Inport
  sfun_PositionActuator : S-Function  FunctionName=sfun_PositionActuator  Parameters=SParameter1, SParameter2, SampleTime  SFunctionDeploymentMode=off  EnableBusSupport=off  mask(Legacy Function){SFunctionSpec=void prescan_outputFcn(void ** work1,  PRESCAN_XYZ_DATA u1[1]), SParameter1=uint8([Object3DID 0]), SParameter2=UniqueID, SampleTime=TimeStep, ShowSpec=on}
      mask prompts: SParameter1 "P1:"; SParameter2 "P2:"; SampleTime "Sample time (-1 for inherited):"; ShowSpec "Display function specification"
      mask help:
      | This block allows you to call the legacy functions specified by the following Legacy Code Tool definition:
      | def.SFunctionName = 'sfun_PositionActuator';
      | def.OutputFcnSpec = 'void prescan_outputFcn(void ** work1,  PRESCAN_XYZ_DATA u1[1])';
      | def.StartFcnSpec = 'void prescan_startFcn(void ** work1, uint8 p1[], double p2)';
      | def.TerminateFcnSpec = 'void prescan_terminateFcn(void ** work1)';
      | def.HeaderFiles = {'prescan_positionactuator_data.h', 'prescan_header_data.h', 'prescan_SFunLibrary.h', 'prescan_CreateLogHandler.h', 'prescan_CreateErrorHandler.h'};
      | def.SourceFiles = {'prescan_MexLogHandler.cpp', 'prescan_SimStructErrorHandler.cpp', 'prescan_ConcurrentLogHandler.cpp', 'prescan_ConcurrentErrorHandler.cpp'};
      | def.HostLibFiles = {'sensorinterfaced.lib'};
      | def.TargetLibFiles = {'sensorinterfaced.so'};
      | def.IncPaths = {'.', 'C:\prescandev\vislibrary\vis\..\pimp\include\sensors\InterfaceRTW'};
      | def.SrcPaths = {'.'};
      | def.LibPaths = {'C:\\prescandev\\vislibrary_build\lib'};
      | def.SampleTime = 'parameterized';
      mask Help: <p>This block was generated automatically by the Legacy Code Tool. For detailed help on this tool, call<a href="matlab:legacy_code('help')"> legacy_code('help')</a>.</p>
      mask Callback ShowSpec:
      | if strcmp(get_param(gcbh, 'ShowSpec'), 'on')
      |   set_param(gcbh, 'MaskDisplay', sprintf('fprintf(''%s'');', get_param(gcbh, 'SFunctionSpec')));
      | else
      |   set_param(gcbh, 'MaskDisplay', sprintf('fprintf(''%s'');', get_param(gcbh, 'FunctionName')));
      | end
      mask Display: fprintf('void prescan_outputFcn(void ** work1,  PRESCAN_XYZ_DATA u1[1])');
  wires:
  In1/1 -> sfun_PositionActuator/1
